simulink model "simulator"  (R2016b)
settings: Solver=ode4  StartTime=0.0  StopTime=10.0  FixedStep=0.01  RelTol=1e-3
InitFcn:
  | parameters
values from neighbouring files (symbols this model uses):
  g = 9.81    [parameters.m]
  I_Q = [Ix Iy Iz].'    [parameters.m]
  l_L = 1.0    (= 1)    [parameters.m]
  m_L = 0.1    [parameters.m]
  m_Q = 1.0    (= 1)    [parameters.m]
  p_S_B = zeros(3,1)    [parameters.m]
  x0_position = x0(1:n/2)    [parameters.m]
  x0_velocity = x0(n/2+1:n)    [parameters.m]
  xf = zeros(n,1)    [parameters.m]
libraries: simulink x1
settings Model: Creator=Youngdong  LastModifiedBy=Youngdong
settings SolverCC: AutoInsertRateTranBlk=on
settings DataIOCC: InitialState=n

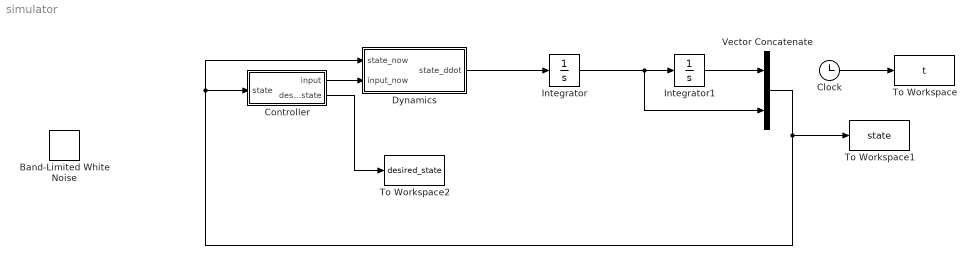
== system simulator ==
  Clock : Clock
  Controller : Subsystem
  Dynamics : Subsystem
  Integrator : Integrator  InitialCondition=x0_velocity
  Integrator1 : Integrator  InitialCondition=x0_position
  To Workspace : ToWorkspace  VariableName=t  SaveFormat=Timeseries  SampleTime=-1
  To Workspace1 : ToWorkspace  VariableName=state  SaveFormat=Timeseries  SampleTime=-1
  To Workspace2 : ToWorkspace  VariableName=desired_state  SaveFormat=Timeseries  SampleTime=-1
  Vector Concatenate : Concatenate
  Band-Limited White Noise : simulink/Sources/Band-Limited White Noise  IOType=siggen  Cov=[0.1]  Ts=0.1  seed=[23341]
  wires:
  Dynamics/1(state_ddot) -> Integrator/1
  Clock/1 -> To Workspace/1
  Integrator/1 -> Vector Concatenate/2, Integrator1/1
  Integrator1/1 -> Vector Concatenate/1
  Vector Concatenate/1 -> Dynamics/1(state_now), Controller/1(state), To Workspace1/1
  Controller/1(input) -> Dynamics/2(input_now)
  Controller/2(desired_state) -> To Workspace2/1

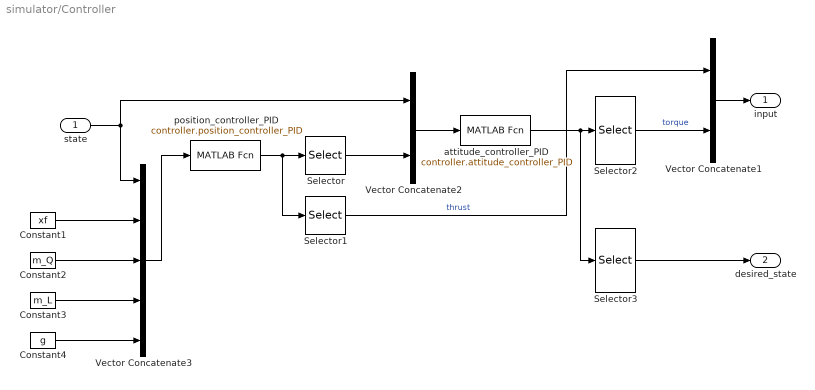
== system simulator/Controller ==
  state : Inport  PortDimensions=n
  Constant1 : Constant  Value=xf
  Constant2 : Constant  Value=m_Q
  Constant3 : Constant  Value=m_L
  Constant4 : Constant  Value=g
  Selector : Selector  InputPortWidth=4  IndexOptions=Index vector (dialog)  Indices=[2 3 4]  OutputSizes=1
  Selector1 : Selector  InputPortWidth=4  IndexOptions=Index vector (dialog)  Indices=[1]  OutputSizes=1
  Selector2 : Selector  InputPortWidth=6  IndexOptions=Index vector (dialog)  Indices=[1 2 3]  OutputSizes=1
  Selector3 : Selector  InputPortWidth=6  IndexOptions=Index vector (dialog)  Indices=[4 5 6]  OutputSizes=1
  Vector Concatenate1 : Concatenate
  Vector Concatenate2 : Concatenate
  Vector Concatenate3 : Concatenate  NumInputs=5
  attitude_controller_PID : MATLABFcn  MATLABFcn=controller.attitude_controller_PID  OutputDimensions=6
  position_controller_PID : MATLABFcn  MATLABFcn=controller.position_controller_PID
  input : Outport  PortDimensions=4
  desired_state : Outport  Port=2  PortDimensions=3
  wires:
  state/1 -> Vector Concatenate3/1, Vector Concatenate2/1
  position_controller_PID/1 -> Selector1/1, Selector/1
  Vector Concatenate1/1 -> input/1
  Selector1/1 -> Vector Concatenate1/1  "thrust"
  Vector Concatenate2/1 -> attitude_controller_PID/1
  Selector/1 -> Vector Concatenate2/2
  Vector Concatenate3/1 -> position_controller_PID/1
  Constant1/1 -> Vector Concatenate3/2
  Constant2/1 -> Vector Concatenate3/3
  Constant3/1 -> Vector Concatenate3/4
  Constant4/1 -> Vector Concatenate3/5
  Selector2/1 -> Vector Concatenate1/2  "torque"
  attitude_controller_PID/1 -> Selector3/1, Selector2/1
  Selector3/1 -> desired_state/1

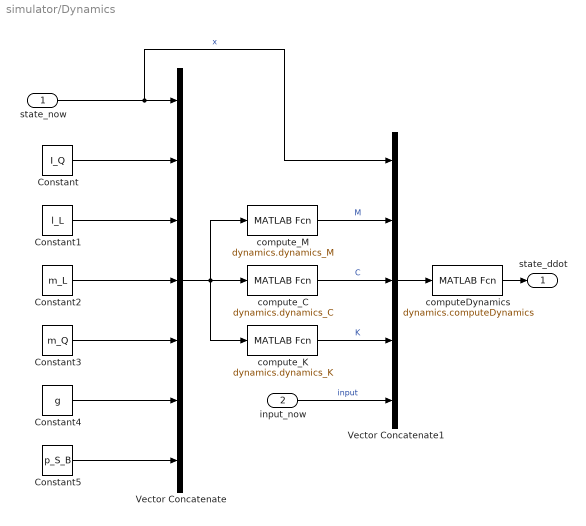
== system simulator/Dynamics ==
  state_now : Inport  PortDimensions=n
  input_now : Inport  Port=2
  Constant : Constant  Value=I_Q
  Constant1 : Constant  Value=l_L
  Constant2 : Constant  Value=m_L
  Constant3 : Constant  Value=m_Q
  Constant4 : Constant  Value=g
  Constant5 : Constant  Value=p_S_B
  Vector Concatenate : Concatenate  NumInputs=7
  Vector Concatenate1 : Concatenate  NumInputs=5
  computeDynamics : MATLABFcn  MATLABFcn=dynamics.computeDynamics  OutputSignalType=real
  compute_C : MATLABFcn  MATLABFcn=dynamics.dynamics_C  OutputSignalType=real
  compute_K : MATLABFcn  MATLABFcn=dynamics.dynamics_K  OutputSignalType=real
  compute_M : MATLABFcn  MATLABFcn=dynamics.dynamics_M  OutputSignalType=real
  state_ddot : Outport
  wires:
  state_now/1 -> Vector Concatenate1/1, Vector Concatenate/1  "x"
  Vector Concatenate1/1 -> computeDynamics/1
  computeDynamics/1 -> state_ddot/1
  compute_M/1 -> Vector Concatenate1/2  "M"
  compute_C/1 -> Vector Concatenate1/3  "C"
  compute_K/1 -> Vector Concatenate1/4  "K"
  Constant/1 -> Vector Concatenate/2
  Constant1/1 -> Vector Concatenate/3
  Constant2/1 -> Vector Concatenate/4
  Constant3/1 -> Vector Concatenate/5
  Constant4/1 -> Vector Concatenate/6
  Constant5/1 -> Vector Concatenate/7
  Vector Concatenate/1 -> compute_K/1, compute_C/1, compute_M/1
  input_now/1 -> Vector Concatenate1/5  "input"
